simulink model "IFOCv6"  (R2022b)
settings: Solver=ode23tb  StartTime=0.0  StopTime=30  MaxStep=1e-5  RelTol=1e-4
InitFcn:
  | IFOCdatav6
values from neighbouring files (symbols this model uses):
  f_n = 300    [FOC_BANG_Script.m]    (also in IFOCdatav6.m)
  Im_n = k_im*Is_n    [FOC_BANG_Script.m]    (also in IFOCdatav6.m)
  Is_n = Pa/(3*Vsn_y*cos_phi)    [FOC_BANG_Script.m]    (also in IFOCdatav6.m)
  J = 5    [Data.m]    (also in FOC_BANG_Script.m; IFOCdatav6.m)
  ki_w = 0.5*(kp_w^2)/J    (= 3.92607044657)    [FOC_BANG_Script.m]    (also in IFOCdatav6.m = 613.448507277)
  kii = (1/2)*kpi^2/Ltot    [IFOCdatav6.m]
  kp_w = T_n/(0.05*wr_n)/5    (= 6.2658362942)    [FOC_BANG_Script.m]    (also in IFOCdatav6.m = 78.3229536775)
  kpi = (1/2)*Ltot/Ts    [IFOCdatav6.m]
  Lm = Phi_n/Im_n    [FOC_BANG_Script.m]    (also in IFOCdatav6.m)
  Lr = Ltot/2    [FOC_BANG_Script.m]    (also in IFOCdatav6.m)
  Ls = Ltot/2    [FOC_BANG_Script.m]    (also in IFOCdatav6.m)
  p = 6    [Data.m]    (also in FOC_BANG_Script.m; IFOCdatav6.m)
  P_n = 150000    [FOC_BANG_Script.m]    (also in IFOCdatav6.m)
  Rr = Rs    [FOC_BANG_Script.m]    (also in IFOCdatav6.m)
  Rs = (Pjs/3)/(Is_n^2)    [FOC_BANG_Script.m]    (also in IFOCdatav6.m)
  sigma_r = Lr/Lm    [FOC_BANG_Script.m]    (also in IFOCdatav6.m)
  sigma_s = Ls/Lm    [FOC_BANG_Script.m]    (also in IFOCdatav6.m)
  T_n = P_n/wr_n    (= 484.735867285)    [FOC_BANG_Script.m]    (also in IFOCdatav6.m)
  Tr = Lm*(1+sigma_r)/Rr    [FOC_BANG_Script.m]    (also in IFOCdatav6.m)
  Ts = 1/fs    (= 5e-05)    [FOC_BANG_Script.m]    (also in IFOCdatav6.m = 0.0001)
  Vdc = 350    [Data.m]    (also in FOC_BANG_Script.m; IFOCdatav6.m)
  Vs_n = 220    [FOC_BANG_Script.m]    (also in IFOCdatav6.m)
  Vsn_y = Vs_n/sqrt(3)    [FOC_BANG_Script.m]    (also in IFOCdatav6.m)
  wr_n = w_n/p*(1-s_n)    (= 309.446876379)    [FOC_BANG_Script.m]    (also in IFOCdatav6.m)
undefined symbols (not defined in the file or in its folder): DiscIntNeverNeededParam, sigbuilder_block
libraries: slpidlib x3, spsControlledVoltageSourceLib x3, spsCurrentMeasurementLib x3, eeTransforms x2, spsAsynchronousMachineSIUnitsLib x1, spsGroundLib x1, simulink x1, sps_lib x1
settings Model: Creator=39388  LastModifiedBy=v4pal
settings DebuggingCC: UnconnectedInputMsg=warning  UnconnectedOutputMsg=warning  UnconnectedLineMsg=warning  SFMachineParentedDataDiag=warning
settings ModelReferenceCC: EnableRefExpFcnMdlSchedulingChecks=on
settings RTWCC: DLArmComputeVersion=19.05

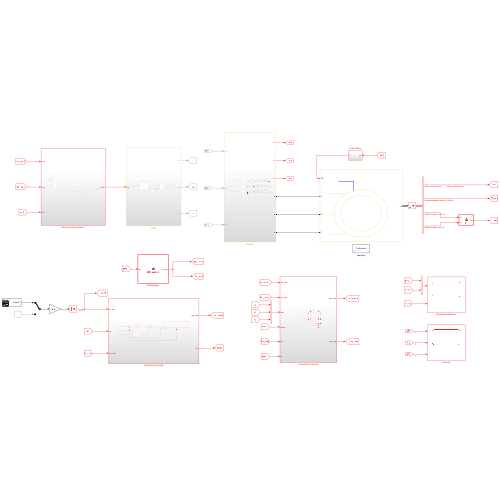
[thumbnail: Simulink's stored preview of the top-level diagram]
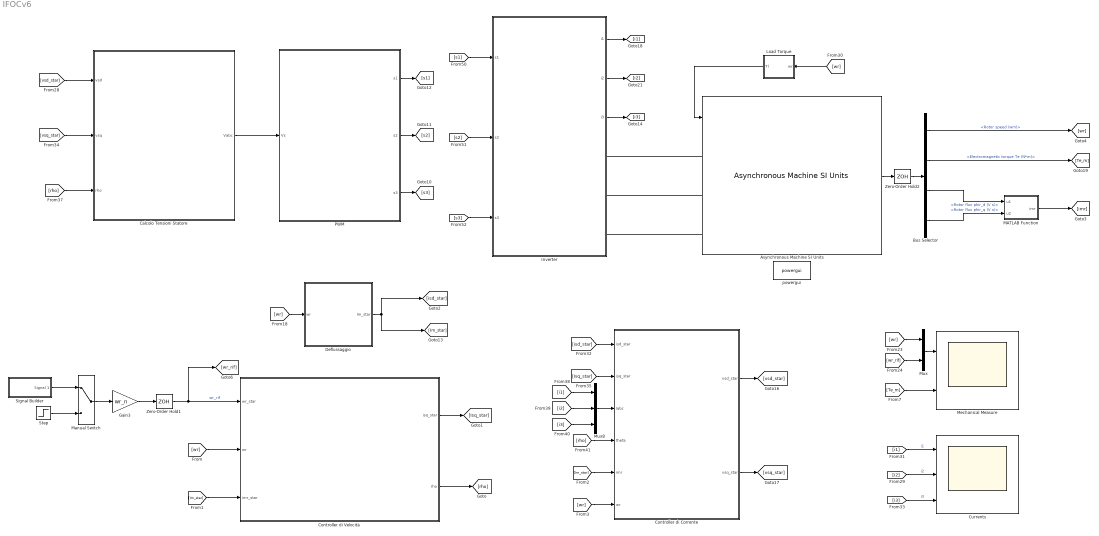
== system IFOCv6 ==
  Asynchronous Machine SI Units : spsAsynchronousMachineSIUnitsLib/Asynchronous Machine SI Units  RotorType=Squirrel-cage  PresetModel=No  MechanicalLoad=Torque Tm  ShowDetailedParameters=on  ReferenceFrame=Rotor  Units=SI  MeasurementBus=off  NominalParameters=[P_n Vs_n f_n]  VoltageRatio=1  Stator=[Rs Ls]  Rotor=[Rr Lr]  Cage1=[0.4155 0.002066]  Cage2=[0.4168 0.0003495]  Lm=Lm  Mechanical=[J 0 p]  PolePairs=2  InitialConditions=[1 0 0 0 0 0 0 0]  SimulateSaturation=off  Saturation=[14.03593122, 27.81365428, 53.79336849, 72.68890987, 97.98006896, 148.6815601, 215.7428561, 302.9841135, 428.7778367 ; 230, 322, 414, 460, 506, 552, 598, 644, 690]  LoadFlowParameters=1492000  TsPowergui=0  TsBlock=-1  IterativeModel=Trapezoidal non iterative  IterativeDiscreteModel=Trapezoidal non iterative  Pmec=1.492e+006
  Bus Selector : BusSelector  OutputSignals=Mechanical.Rotor speed (wm),Mechanical.Electromagnetic torque Te (N*m),Rotor measurements.Rotor flux phir_d (V s),Rotor measurements.Rotor flux phir_q (V s)
  "Calcolo Tensioni Statore " : Subsystem
  Controller di Corrente : Subsystem
  Controller di Velocità : Subsystem
  Currents : Scope  NumInputPorts=3
  Deflussaggio : MATLAB Function  TreatAsAtomicUnit=on
  Gain3 : Gain  Gain=wr_n
  Inverter : Subsystem
  Load Torque : Subsystem
  MATLAB Function : MATLAB Function  TreatAsAtomicUnit=on
  Manual Switch : ManualSwitch
  Mechanical Measure : Scope  NumInputPorts=2
  Mux : Mux  Inputs=2
  Mux8 : Mux  Inputs=3
  PWM : Subsystem
  Signal Builder : Subsystem  Tag=STV Subsys  LoadFcn=sigbuilder_block('load');  StartFcn=sigbuilder_block('start');  StopFcn=sigbuilder_block('stop');  ClipboardFcn=sigbuilder_block('clipboard');  mask(Sigbuilder block){tuvar=[0:10]}
      mask help: Simulink:masks:SigbuilderBlock_MD
      mask init:
      | if ~strcmp(get_param(bdroot(gcbh),'SimulationStatus'),'stopped') tuvar = sigbuilder_block('maskInit'); end
      settings: CopyFcn=sigbuilder_block('copy');  DeleteFcn=sigbuilder_block('delete');  ModelCloseFcn=sigbuilder_block('modelClose');  PreSaveFcn=sigbuilder_block('preSave');  PauseFcn=sigbuilder_block('pause');  ContinueFcn=sigbuilder_block('continue');  NameChangeFcn=sigbuilder_block('namechange');  OpenFcn=sigbuilder_block('open',[433.2 162 550.8 400.2 ]);  CloseFcn=sigbuilder_block('close');
      mask Display: plot(0, 0, 100, 100,[2, 2, 32, 32, 2], [68, 8, 8, 68, 68],[32, 2], [38, 38], [32, 19, 2],[53, 60, 44], [32, 17, 17, 2],[16, 16, 31, 31]);txt = getActiveGroup(gcbh);text(2, 100, txt,'verticalAlignment', 'top');
  Step : Step  Time=0  After=2  SampleTime=0
  Zero-Order Hold1 : ZeroOrderHold  SampleTime=Ts
  Zero-Order Hold2 : ZeroOrderHold  SampleTime=Ts
  powergui : sps_lib/powergui  Priority=1  SimulationMode=Continuous  SampleTime=50e-6  frequency=60  Iterations=50  frequencyindice=0  Pbase=100e6  ErrMax=1e-4  UnitsV=kV  UnitsW=MW  buscounter=0  FunctionMessages=off  echomessages=off  EnableUseOfTLC=off  CurrentSourceSwitches=off  DisableSnubberDevices=off  DisableRonSwitches=off  DisableVfSwitches=off  DisplayEquations=off  AutomaticDiscreteSolvers=off  SolverType=Tustin/Backward Euler (TBE)  Interpol=off  ExternalGateDelay=off  methode=off  Ts=100  x0status=blocks  SPID=on  SwTol=0  HookPort=off  NonlinearTolerance=1e-4  nMaxIteration=100  ContinueOnMaxIteration=off  RestoreLinks=warning  ResistiveCurrentMeasurement=off  Frange=[0:2:500]  Ylog=off  Xlog=on  ShowGrid=off  save=off  variable=ZData  structure=0  ZoomFFT=off  StartTime=0.0  cycles=1  DisplayStyle=1  fundamental=60  FreqAxis=off  MaxFrequency=1000  frequencyindicesteady=1  RmsSteady=1  display=off
  wires:
  Asynchronous Machine SI Units/1 -> Zero-Order Hold2/1
  Bus Selector/1 -> [wr]  "<Rotor speed (wm)>"
  [wr] -> Load Torque/1(wr)
  Load Torque/1(Tl) -> Asynchronous Machine SI Units/1
  [wr] -> Deflussaggio/1(wr)
  Zero-Order Hold1/1 -> [wr_rif], Controller di Velocità/1(wr_star)  "wr_rif"
  Gain3/1 -> Zero-Order Hold1/1
  Manual Switch/1 -> Gain3/1
  Signal Builder/1(Signal 1) -> Manual Switch/1
  Step/1 -> Manual Switch/2
  [i2] -> Currents/2  "i2"
  [i3] -> Currents/3  "i3"
  [i1] -> Currents/1  "i1"
  [i1] -> Mux8/1
  [i3] -> Mux8/3
  [i2] -> Mux8/2
  Bus Selector/2 -> [Te_m]  "<Electromagnetic torque Te (N*m)>"
  Deflussaggio/1(Im_star) -> [isd_star], [Im_star]
  PWM/1(s1) -> [s1]
  PWM/2(s2) -> [s2]
  PWM/3(s3) -> [s3]
  [vsd_star] -> "Calcolo Tensioni Statore "/1(vsd)
  [vsq_star] -> "Calcolo Tensioni Statore "/2(vsq)
  [rho] -> "Calcolo Tensioni Statore "/3(rho)
  [isd_star] -> Controller di Corrente/1(isd_star)
  [Isq_star] -> Controller di Corrente/2(isq_star)
  Mux8/1 -> Controller di Corrente/3(Iabc)
  [rho] -> Controller di Corrente/4(theta)
  Controller di Corrente/1(vsd_star) -> [vsd_star]
  Controller di Corrente/2(vsq_star) -> [vsq_star]
  [wr] -> Controller di Velocità/2(wr)
  [Im_star] -> Controller di Velocità/3(imr_star)
  Controller di Velocità/1(isq_star) -> [Isq_star]
  Controller di Velocità/2(rho) -> [rho]
  [s1] -> Inverter/1(s1)
  [s2] -> Inverter/2(s2)
  [s3] -> Inverter/3(s3)
  Inverter/1(i1) -> [i1]
  Inverter/2(i2) -> [i2]
  Inverter/3(i3) -> [i3]
  Bus Selector/3 -> MATLAB Function/1(u1)  "<Rotor flux phir_d (V s)>"
  Bus Selector/4 -> MATLAB Function/2(u2)  "<Rotor flux phir_q (V s)>"
  MATLAB Function/1(imr) -> [imr]
  "Calcolo Tensioni Statore "/1(Vabc) -> PWM/1(Vs)
  [Im_star] -> Controller di Corrente/5(imr)
  Zero-Order Hold2/1 -> Bus Selector/1
  [wr] -> Controller di Corrente/6(wr)
  [Te_m] -> Mechanical Measure/2
  Mux/1 -> Mechanical Measure/1
  [wr] -> Mux/1
  [wr_rif] -> Mux/2
  connections:
  Asynchronous Machine SI Units/LConn1 -- Inverter/RConn1
  Asynchronous Machine SI Units/LConn2 -- Inverter/RConn2
  Asynchronous Machine SI Units/LConn3 -- Inverter/RConn3

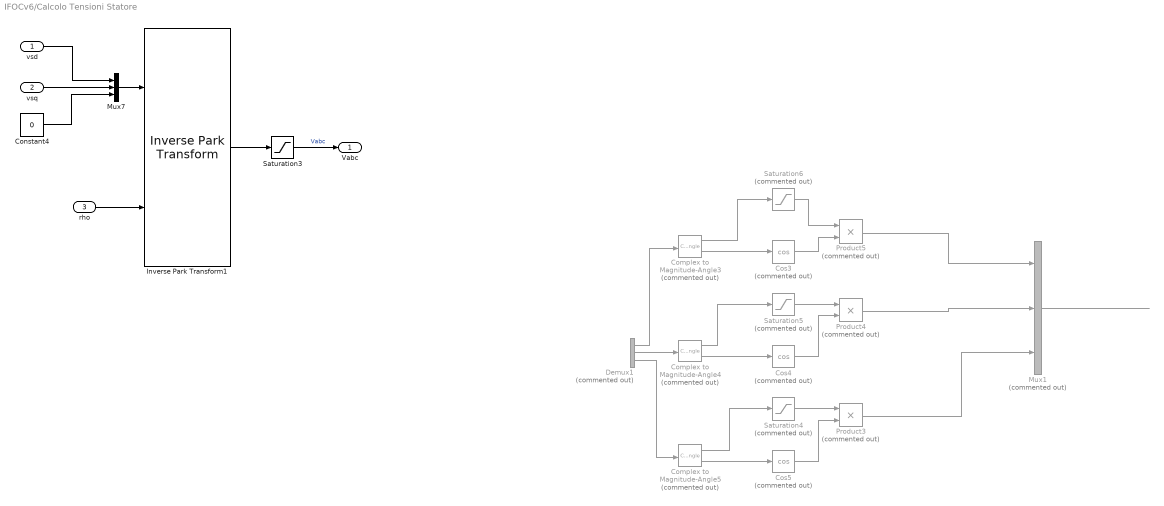
== system IFOCv6/Calcolo Tensioni Statore  ==
  vsd : Inport
  vsq : Inport  Port=2
  rho : Inport  Port=3
  Complex to Magnitude-Angle3 : ComplexToMagnitudeAngle  Commented=on
  Complex to Magnitude-Angle4 : ComplexToMagnitudeAngle  Commented=on
  Complex to Magnitude-Angle5 : ComplexToMagnitudeAngle  Commented=on
  Constant4 : Constant  Value=0
  Cos3 : Trigonometry  Commented=on  Operator=cos
  Cos4 : Trigonometry  Commented=on  Operator=cos
  Cos5 : Trigonometry  Commented=on  Operator=cos
  Demux1 : Demux  Commented=on  Outputs=3
  Inverse Park Transform1 : eeTransforms/Inverse Park Transform  AxisAlignment=Q-axis  PowerInvariant=off
      settings: LibrarySourceBlock=|
      | ee_sl_lib/Mathematical
      | Transforms/Inverse
      | Park Transform
  Mux1 : Mux  Commented=on  Inputs=3
  Mux7 : Mux  Inputs=3
  Product3 : Product  Commented=on
  Product4 : Product  Commented=on
  Product5 : Product  Commented=on
  Saturation3 : Saturate  UpperLimit=Vsn_y*sqrt(2)  LowerLimit=-Vsn_y*sqrt(2)
  Saturation4 : Saturate  Commented=on  UpperLimit=Vsn_y*sqrt(2)  LowerLimit=-Vsn_y*sqrt(2)
  Saturation5 : Saturate  Commented=on  UpperLimit=Vsn_y*sqrt(2)  LowerLimit=-Vsn_y*sqrt(2)
  Saturation6 : Saturate  Commented=on  UpperLimit=Vsn_y*sqrt(2)  LowerLimit=-Vsn_y*sqrt(2)
  Vabc : Outport
  wires:
  Mux7/1 -> Inverse Park Transform1/1
  Constant4/1 -> Mux7/3
  vsd/1 -> Mux7/1
  vsq/1 -> Mux7/2
  rho/1 -> Inverse Park Transform1/2
  Saturation6/1 -> Product5/1
  Saturation5/1 -> Product4/1
  Saturation4/1 -> Product3/1
  Complex to Magnitude-Angle5/1 -> Saturation4/1
  Complex to Magnitude-Angle3/1 -> Saturation6/1
  Cos3/1 -> Product5/2
  Complex to Magnitude-Angle4/1 -> Saturation5/1
  Cos4/1 -> Product4/2
  Cos5/1 -> Product3/2
  Complex to Magnitude-Angle5/2 -> Cos5/1
  Complex to Magnitude-Angle4/2 -> Cos4/1
  Complex to Magnitude-Angle3/2 -> Cos3/1
  Product3/1 -> Mux1/3
  Product4/1 -> Mux1/2
  Product5/1 -> Mux1/1
  Demux1/3 -> Complex to Magnitude-Angle5/1
  Demux1/2 -> Complex to Magnitude-Angle4/1
  Demux1/1 -> Complex to Magnitude-Angle3/1
  ? -> Demux1/1
  Mux1/1 -> ?
  Inverse Park Transform1/1 -> Saturation3/1
  Saturation3/1 -> Vabc/1  "Vabc"

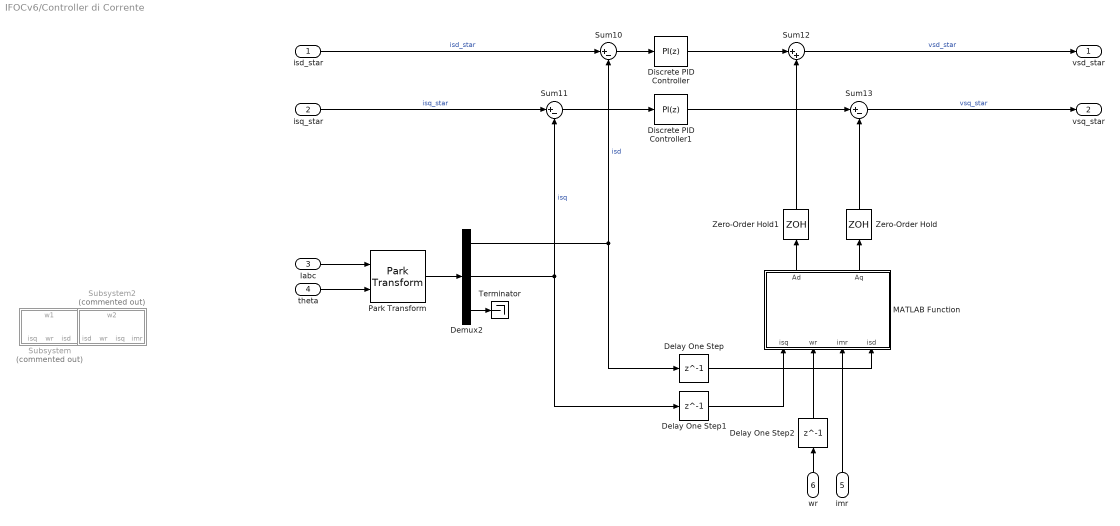
== system IFOCv6/Controller di Corrente ==
  isd_star : Inport
  isq_star : Inport  Port=2
  Iabc : Inport  Port=3
  theta : Inport  Port=4
  imr : Inport  Port=5
  wr : Inport  Port=6
  Delay One Step : Delay  DelayLength=1
  Delay One Step1 : Delay  DelayLength=1  InitialCondition=Im_n
  Delay One Step2 : Delay  DelayLength=1
  Demux2 : Demux  Outputs=3
  Discrete PID Controller : slpidlib/PID Controller  Controller=PI  Form=Parallel  TimeDomain=Discrete-time  UseExternalTs=off  SampleTime=Ts  IntegratorMethod=Forward Euler  FilterMethod=Forward Euler  ControllerParametersSource=internal  P=kpi  I=0.5*kii  UseKiTs=off  D=0  N=100  UseFilter=on  TunerSelectOption=Transfer Function Based (PID Tuner App)  InitialConditionSource=internal  InitialConditionForIntegrator=0  InitialConditionForFilter=0  DifferentiatorICPrevScaledInput=0  ExternalReset=none  TrackingMode=off  Kt=1  LimitOutput=on  SatLimitsSource=internal  UpperSaturationLimit=inf  LowerSaturationLimit=-inf  LinearizeAsGain=off  AntiWindupMode=clamping  Kb=1  LimitIntegrator=off  UpperIntegratorSaturationLimit=inf  LowerIntegratorSaturationLimit=-inf  POutMin=[]  POutMax=[]  IOutMin=[]  IOutMax=[]  DOutMin=[]  DOutMax=[]  NOutMin=[]  NOutMax=[]  SumOutMin=[]  SumOutMax=[]  SaturationOutMin=[]  SaturationOutMax=[]  PParamMin=[]  PParamMax=[]  IParamMin=[]  IParamMax=[]  DParamMin=[]  DParamMax=[]  NParamMin=[]  NParamMax=[]  KbParamMin=[]  KbParamMax=[]  KtParamMin=[]  KtParamMax=[]  KbOutMin=[]  KbOutMax=[]  KtOutMin=[]  KtOutMax=[]  IntegratorOutMin=[]  IntegratorOutMax=[]  FilterOutMin=[]  FilterOutMax=[]  SumI1OutMin=[]  SumI1OutMax=[]  SumI2OutMin=[]  SumI2OutMax=[]  SumI3OutMin=[]  SumI3OutMax=[]  SumI4OutMin=[]  SumI4OutMax=[]  SumDOutMin=[]  SumDOutMax=[]  DifferentiatorOutMin=[]  DifferentiatorOutMax=[]  FilterDiffOutCoefMin=[]  FilterDiffOutCoefMax=[]  ReciprocalOutMin=[]  ReciprocalOutMax=[]  SumDenOutMin=[]  SumDenOutMax=[]  SumNumOutMin=[]  SumNumOutMax=[]  DivideOutMin=[]  DivideOutMax=[]  UdiffTsProdOutMin=[]  UdiffTsProdOutMax=[]  NTsProdOutMin=[]  NTsProdOutMax=[]  UintegralTsProdOutMin=[]  UintegralTsProdOutMax=[]  UngainTsProdOutMin=[]  UngainTsProdOutMax=[]  ClampingZeroOutDataTypeStr=Inherit: Inherit via back propagation  ClampingZeroOutMin=[]  ClampingZeroOutMax=[]  FilterDenConstantOutDataTypeStr=Inherit: Inherit via back propagation  FilterDenConstantOutMin=[]  FilterDenConstantOutMax=[]  PCopyOutDataTypeStr=Inherit: Inherit via back propagation  PCopyOutMin=[]  PCopyOutMax=[]  NCopyOutDataTypeStr=Inherit: Inherit via back propagation  NCopyOutMin=[]  NCopyOutMax=[]  IntegratorContinuousStateAttributes=''  IntegratorStateMustResolveToSignalObject=off  IntegratorRTWStateStorageClass=Auto  FilterContinuousStateAttributes=''  FilterStateMustResolveToSignalObject=off  FilterRTWStateStorageClass=Auto  ParallelPVariant=InternalParameters  IdealPVariant=Disabled  IVariant=InternalParameters  DVariant=Disabled  IntegratorVariant=Discrete  SatVariant=Enabled  AWVariant=DiscClampingParallel  PCopyVariant=Disabled  TRVariant=Disabled  FdbkBlocksVariant=Forward  IdealPFdbkVariant=Disabled  SatFdbkVariant=Disabled  DerivativeFilterVariant=Disabled  NVariant=Disabled  NCopyVariant=Disabled_SignalSpec  FilterICVariant=Disabled  IntegratorICVariant=InternalICs  ExternalResetVariant=Disabled  TRSumVariant=Passthrough  SumFdbkVariant=Disabled  SumVariant=Sum_PI  TsampFilterVariant=InternalTs  TsampNgainVariant=Passthrough  TsampIntegralVariant=Passthrough  ExternalSaturationOutDataTypeStr=Inherit: Same as second input
      settings: LibrarySourceBlock=simulink/Discrete/Discrete PID Controller
  Discrete PID Controller1 : slpidlib/PID Controller  Controller=PI  Form=Parallel  TimeDomain=Discrete-time  UseExternalTs=off  SampleTime=Ts  IntegratorMethod=Forward Euler  FilterMethod=Forward Euler  ControllerParametersSource=internal  P=kpi  I=0.5*kii  UseKiTs=off  D=0  N=100  UseFilter=on  TunerSelectOption=Transfer Function Based (PID Tuner App)  InitialConditionSource=internal  InitialConditionForIntegrator=0  InitialConditionForFilter=0  DifferentiatorICPrevScaledInput=0  ExternalReset=none  TrackingMode=off  Kt=1  LimitOutput=on  SatLimitsSource=internal  UpperSaturationLimit=inf  LowerSaturationLimit=-inf  LinearizeAsGain=off  AntiWindupMode=clamping  Kb=1  LimitIntegrator=off  UpperIntegratorSaturationLimit=inf  LowerIntegratorSaturationLimit=-inf  POutMin=[]  POutMax=[]  IOutMin=[]  IOutMax=[]  DOutMin=[]  DOutMax=[]  NOutMin=[]  NOutMax=[]  SumOutMin=[]  SumOutMax=[]  SaturationOutMin=[]  SaturationOutMax=[]  PParamMin=[]  PParamMax=[]  IParamMin=[]  IParamMax=[]  DParamMin=[]  DParamMax=[]  NParamMin=[]  NParamMax=[]  KbParamMin=[]  KbParamMax=[]  KtParamMin=[]  KtParamMax=[]  KbOutMin=[]  KbOutMax=[]  KtOutMin=[]  KtOutMax=[]  IntegratorOutMin=[]  IntegratorOutMax=[]  FilterOutMin=[]  FilterOutMax=[]  SumI1OutMin=[]  SumI1OutMax=[]  SumI2OutMin=[]  SumI2OutMax=[]  SumI3OutMin=[]  SumI3OutMax=[]  SumI4OutMin=[]  SumI4OutMax=[]  SumDOutMin=[]  SumDOutMax=[]  DifferentiatorOutMin=[]  DifferentiatorOutMax=[]  FilterDiffOutCoefMin=[]  FilterDiffOutCoefMax=[]  ReciprocalOutMin=[]  ReciprocalOutMax=[]  SumDenOutMin=[]  SumDenOutMax=[]  SumNumOutMin=[]  SumNumOutMax=[]  DivideOutMin=[]  DivideOutMax=[]  UdiffTsProdOutMin=[]  UdiffTsProdOutMax=[]  NTsProdOutMin=[]  NTsProdOutMax=[]  UintegralTsProdOutMin=[]  UintegralTsProdOutMax=[]  UngainTsProdOutMin=[]  UngainTsProdOutMax=[]  ClampingZeroOutDataTypeStr=Inherit: Inherit via back propagation  ClampingZeroOutMin=[]  ClampingZeroOutMax=[]  FilterDenConstantOutDataTypeStr=Inherit: Inherit via back propagation  FilterDenConstantOutMin=[]  FilterDenConstantOutMax=[]  PCopyOutDataTypeStr=Inherit: Inherit via back propagation  PCopyOutMin=[]  PCopyOutMax=[]  NCopyOutDataTypeStr=Inherit: Inherit via back propagation  NCopyOutMin=[]  NCopyOutMax=[]  IntegratorContinuousStateAttributes=''  IntegratorStateMustResolveToSignalObject=off  IntegratorRTWStateStorageClass=Auto  FilterContinuousStateAttributes=''  FilterStateMustResolveToSignalObject=off  FilterRTWStateStorageClass=Auto  ParallelPVariant=InternalParameters  IdealPVariant=Disabled  IVariant=InternalParameters  DVariant=Disabled  IntegratorVariant=Discrete  SatVariant=Enabled  AWVariant=DiscClampingParallel  PCopyVariant=Disabled  TRVariant=Disabled  FdbkBlocksVariant=Forward  IdealPFdbkVariant=Disabled  SatFdbkVariant=Disabled  DerivativeFilterVariant=Disabled  NVariant=Disabled  NCopyVariant=Disabled_SignalSpec  FilterICVariant=Disabled  IntegratorICVariant=InternalICs  ExternalResetVariant=Disabled  TRSumVariant=Passthrough  SumFdbkVariant=Disabled  SumVariant=Sum_PI  TsampFilterVariant=InternalTs  TsampNgainVariant=Passthrough  TsampIntegralVariant=Passthrough  ExternalSaturationOutDataTypeStr=Inherit: Same as second input
      settings: LibrarySourceBlock=simulink/Discrete/Discrete PID Controller
  MATLAB Function : MATLAB Function  TreatAsAtomicUnit=on
  Park Transform : eeTransforms/Park Transform  AxisAlignment=Q-axis  PowerInvariant=off
      settings: LibrarySourceBlock=|
      | ee_sl_lib/Mathematical
      | Transforms/Park Transform
  Subsystem : Subsystem  Commented=on
  Subsystem2 : Subsystem  Commented=on
  Sum10 : Sum  Inputs=|+-
  Sum11 : Sum  Inputs=|+-
  Sum12 : Sum  Inputs=|++
  Sum13 : Sum  Inputs=|+-
  Terminator : Terminator
  Zero-Order Hold : ZeroOrderHold  SampleTime=-1
  Zero-Order Hold1 : ZeroOrderHold  SampleTime=-1
  vsd_star : Outport
  vsq_star : Outport  Port=2
  wires:
  Sum13/1 -> vsq_star/1  "vsq_star"
  Park Transform/1 -> Demux2/1
  Demux2/2 -> Delay One Step1/1, Sum11/2  "isq"
  Demux2/1 -> Delay One Step/1, Sum10/2  "isd"
  Sum12/1 -> vsd_star/1  "vsd_star"
  Sum10/1 -> Discrete PID Controller/1
  Sum11/1 -> Discrete PID Controller1/1
  Demux2/3 -> Terminator/1
  isq_star/1 -> Sum11/1  "isq_star"
  theta/1 -> Park Transform/2
  Iabc/1 -> Park Transform/1
  isd_star/1 -> Sum10/1  "isd_star"
  Discrete PID Controller1/1 -> Sum13/1
  Discrete PID Controller/1 -> Sum12/1
  Zero-Order Hold/1 -> Sum13/2
  Zero-Order Hold1/1 -> Sum12/2
  MATLAB Function/2(Aq) -> Zero-Order Hold/1
  MATLAB Function/1(Ad) -> Zero-Order Hold1/1
  Delay One Step/1 -> MATLAB Function/4(isd)
  Delay One Step1/1 -> MATLAB Function/1(isq)
  Delay One Step2/1 -> MATLAB Function/2(wr)
  imr/1 -> MATLAB Function/3(imr)
  wr/1 -> Delay One Step2/1

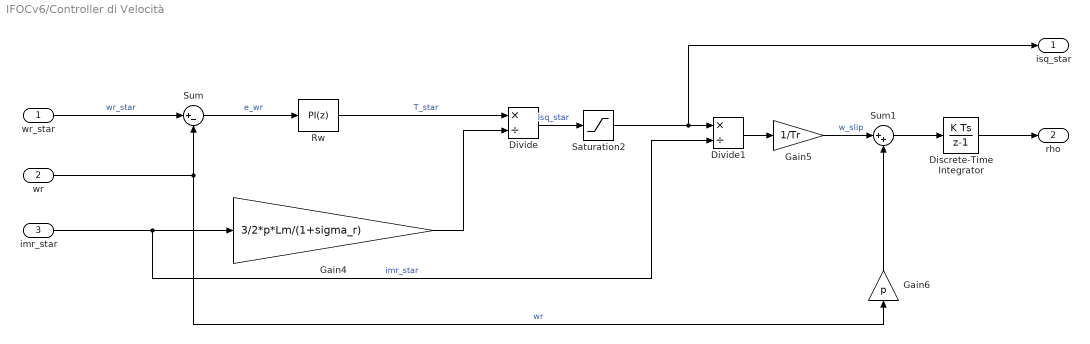
== system IFOCv6/Controller di Velocità ==
  wr_star : Inport
  wr : Inport  Port=2
  imr_star : Inport  Port=3
  Discrete-Time Integrator : DiscreteIntegrator  SampleTime=Ts  ICPrevOutput=DiscIntNeverNeededParam  ICPrevScaledInput=DiscIntNeverNeededParam
  Divide : Product  Inputs=*/
  Divide1 : Product  Inputs=*/
  Gain4 : Gain  Gain=3/2*p*Lm/(1+sigma_r)
  Gain5 : Gain  Gain=1/Tr
  Gain6 : Gain  Gain=p
  Rw : slpidlib/PID Controller  Controller=PI  Form=Parallel  TimeDomain=Discrete-time  UseExternalTs=off  SampleTime=Ts  IntegratorMethod=Trapezoidal  FilterMethod=Forward Euler  ControllerParametersSource=internal  P=kp_w  I=ki_w  UseKiTs=off  D=0  N=100  UseFilter=on  TunerSelectOption=Frequency Response Based  InitialConditionSource=internal  InitialConditionForIntegrator=0  InitialConditionForFilter=0  DifferentiatorICPrevScaledInput=0  ExternalReset=none  TrackingMode=off  Kt=1  LimitOutput=on  SatLimitsSource=internal  UpperSaturationLimit=T_n  LowerSaturationLimit=-T_n  LinearizeAsGain=on  AntiWindupMode=clamping  Kb=1  LimitIntegrator=off  UpperIntegratorSaturationLimit=inf  LowerIntegratorSaturationLimit=-inf  POutMin=[]  POutMax=[]  IOutMin=[]  IOutMax=[]  DOutMin=[]  DOutMax=[]  NOutMin=[]  NOutMax=[]  SumOutMin=[]  SumOutMax=[]  SaturationOutMin=[]  SaturationOutMax=[]  PParamMin=[]  PParamMax=[]  IParamMin=[]  IParamMax=[]  DParamMin=[]  DParamMax=[]  NParamMin=[]  NParamMax=[]  KbParamMin=[]  KbParamMax=[]  KtParamMin=[]  KtParamMax=[]  KbOutMin=[]  KbOutMax=[]  KtOutMin=[]  KtOutMax=[]  IntegratorOutMin=[]  IntegratorOutMax=[]  FilterOutMin=[]  FilterOutMax=[]  SumI1OutMin=[]  SumI1OutMax=[]  SumI2OutMin=[]  SumI2OutMax=[]  SumI3OutMin=[]  SumI3OutMax=[]  SumI4OutMin=[]  SumI4OutMax=[]  SumDOutMin=[]  SumDOutMax=[]  DifferentiatorOutMin=[]  DifferentiatorOutMax=[]  FilterDiffOutCoefMin=[]  FilterDiffOutCoefMax=[]  ReciprocalOutMin=[]  ReciprocalOutMax=[]  SumDenOutMin=[]  SumDenOutMax=[]  SumNumOutMin=[]  SumNumOutMax=[]  DivideOutMin=[]  DivideOutMax=[]  UdiffTsProdOutMin=[]  UdiffTsProdOutMax=[]  NTsProdOutMin=[]  NTsProdOutMax=[]  UintegralTsProdOutMin=[]  UintegralTsProdOutMax=[]  UngainTsProdOutMin=[]  UngainTsProdOutMax=[]  ClampingZeroOutDataTypeStr=Inherit: Inherit via back propagation  ClampingZeroOutMin=[]  ClampingZeroOutMax=[]  FilterDenConstantOutDataTypeStr=Inherit: Inherit via back propagation  FilterDenConstantOutMin=[]  FilterDenConstantOutMax=[]  PCopyOutDataTypeStr=Inherit: Inherit via back propagation  PCopyOutMin=[]  PCopyOutMax=[]  NCopyOutDataTypeStr=Inherit: Inherit via back propagation  NCopyOutMin=[]  NCopyOutMax=[]  IntegratorContinuousStateAttributes=''  IntegratorStateMustResolveToSignalObject=off  IntegratorRTWStateStorageClass=Auto  FilterContinuousStateAttributes=''  FilterStateMustResolveToSignalObject=off  FilterRTWStateStorageClass=Auto  ParallelPVariant=InternalParameters  IdealPVariant=Disabled  IVariant=InternalParameters  DVariant=Disabled  IntegratorVariant=Discrete  SatVariant=Enabled  AWVariant=DiscClampingParallel  PCopyVariant=Disabled  TRVariant=Disabled  FdbkBlocksVariant=Feedback  IdealPFdbkVariant=Passthrough  SatFdbkVariant=Passthrough  DerivativeFilterVariant=Disabled  NVariant=Disabled  NCopyVariant=Disabled_SignalSpec  FilterICVariant=Disabled  IntegratorICVariant=InternalICs  ExternalResetVariant=Disabled  TRSumVariant=Passthrough  SumFdbkVariant=Enabled  SumVariant=Sum_PI  TsampFilterVariant=InternalTs  TsampNgainVariant=Passthrough  TsampIntegralVariant=Passthrough  ExternalSaturationOutDataTypeStr=Inherit: Same as second input
  Saturation2 : Saturate  UpperLimit=0.96*Is_n*sqrt(2)  LowerLimit=-0.96*Is_n*sqrt(2)
  Sum : Sum  Inputs=|+-
  Sum1 : Sum  Inputs=|++
  isq_star : Outport
  rho : Outport  Port=2
  wires:
  Sum1/1 -> Discrete-Time Integrator/1
  Divide1/1 -> Gain5/1
  Gain5/1 -> Sum1/1  "w_slip"
  Gain6/1 -> Sum1/2
  wr/1 -> Gain6/1, Sum/2  "wr"
  Sum/1 -> Rw/1  "e_wr"
  Rw/1 -> Divide/1  "T_star"
  Gain4/1 -> Divide/2
  Divide/1 -> Saturation2/1  "Isq_star"
  wr_star/1 -> Sum/1  "wr_star"
  Discrete-Time Integrator/1 -> rho/1
  imr_star/1 -> Divide1/2, Gain4/1  "imr_star"
  Saturation2/1 -> isq_star/1, Divide1/1

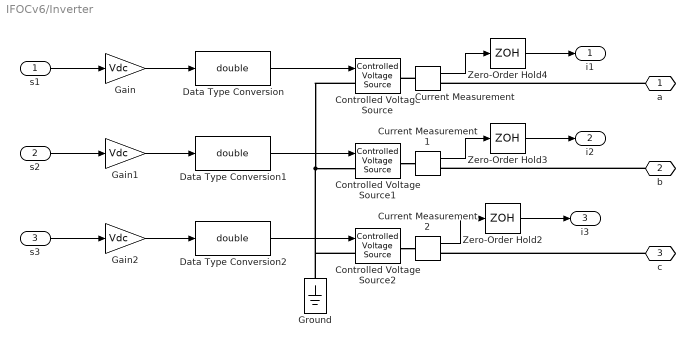
== system IFOCv6/Inverter ==
  s1 : Inport
  s2 : Inport  Port=2
  s3 : Inport  Port=3
  Controlled Voltage Source : spsControlledVoltageSourceLib/Controlled Voltage Source  Initialize=on  Source_Type=AC  Amplitude=0  Phase=0  Frequency=0  Measurements=None
  Controlled Voltage Source1 : spsControlledVoltageSourceLib/Controlled Voltage Source  Initialize=on  Source_Type=AC  Amplitude=0  Phase=0  Frequency=0  Measurements=None
  Controlled Voltage Source2 : spsControlledVoltageSourceLib/Controlled Voltage Source  Initialize=on  Source_Type=AC  Amplitude=0  Phase=0  Frequency=0  Measurements=None
  Current Measurement : spsCurrentMeasurementLib/Current Measurement  PhasorSimulation=off  OutputType=Complex  PSBequivalent=0
  Current Measurement1 : spsCurrentMeasurementLib/Current Measurement  PhasorSimulation=off  OutputType=Complex  PSBequivalent=0
  Current Measurement2 : spsCurrentMeasurementLib/Current Measurement  PhasorSimulation=off  OutputType=Complex  PSBequivalent=0
  Data Type Conversion : DataTypeConversion  OutDataTypeStr=double  SaturateOnIntegerOverflow=off  RndMeth=Floor
  Data Type Conversion1 : DataTypeConversion  OutDataTypeStr=double  SaturateOnIntegerOverflow=off  RndMeth=Floor
  Data Type Conversion2 : DataTypeConversion  OutDataTypeStr=double  SaturateOnIntegerOverflow=off  RndMeth=Floor
  Gain : Gain  Gain=Vdc
  Gain1 : Gain  Gain=Vdc
  Gain2 : Gain  Gain=Vdc
  Ground : spsGroundLib/Ground  LConnTagsString=a
  Zero-Order Hold2 : ZeroOrderHold  SampleTime=Ts
  Zero-Order Hold3 : ZeroOrderHold  SampleTime=Ts
  Zero-Order Hold4 : ZeroOrderHold  SampleTime=Ts
  a : PMIOPort  Side=Right
  b : PMIOPort  Port=2  Side=Right
  c : PMIOPort  Port=3  Side=Right
  i1 : Outport
  i2 : Outport  Port=2
  i3 : Outport  Port=3
  wires:
  Gain/1 -> Data Type Conversion/1
  Zero-Order Hold4/1 -> i1/1
  Gain1/1 -> Data Type Conversion1/1
  Current Measurement2/1 -> Zero-Order Hold2/1
  Current Measurement/1 -> Zero-Order Hold4/1
  Gain2/1 -> Data Type Conversion2/1
  Current Measurement1/1 -> Zero-Order Hold3/1
  Data Type Conversion1/1 -> Controlled Voltage Source1/1
  Data Type Conversion2/1 -> Controlled Voltage Source2/1
  s3/1 -> Gain2/1
  Data Type Conversion/1 -> Controlled Voltage Source/1
  s2/1 -> Gain1/1
  Zero-Order Hold2/1 -> i3/1
  Zero-Order Hold3/1 -> i2/1
  s1/1 -> Gain/1
  connections:
  Controlled Voltage Source/LConn1 -- Ground/LConn1 -- Controlled Voltage Source2/LConn1 -- Controlled Voltage Source1/LConn1
  Controlled Voltage Source1/RConn1 -- Current Measurement1/LConn1
  Controlled Voltage Source2/RConn1 -- Current Measurement2/LConn1
  Current Measurement/LConn1 -- Controlled Voltage Source/RConn1
  b/RConn1 -- Current Measurement1/RConn1
  a/RConn1 -- Current Measurement/RConn1
  c/RConn1 -- Current Measurement2/RConn1

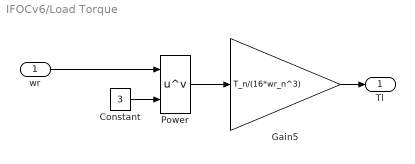
== system IFOCv6/Load Torque ==
  wr : Inport
  Constant : Constant  Value=3
  Gain5 : Gain  Gain=T_n/(16*wr_n^3)
  Power : Math  Operator=pow
  Tl : Outport
  wires:
  Power/1 -> Gain5/1
  Constant/1 -> Power/2
  Gain5/1 -> Tl/1
  wr/1 -> Power/1

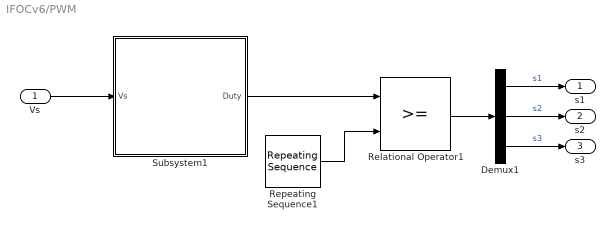
== system IFOCv6/PWM ==
  Vs : Inport
  Demux1 : Demux  Outputs=3
  Relational Operator1 : RelationalOperator  OutDataTypeStr=boolean  RndMeth=Simplest  InputSameDT=off
  Repeating Sequence1 : simulink/Sources/Repeating Sequence  rep_seq_t=[0 Ts/2 Ts]  rep_seq_y=[0 1 0]
  Subsystem1 : Subsystem
  s1 : Outport
  s2 : Outport  Port=2
  s3 : Outport  Port=3
  wires:
  Vs/1 -> Subsystem1/1(Vs)
  Subsystem1/1(Duty) -> Relational Operator1/1
  Repeating Sequence1/1 -> Relational Operator1/2
  Demux1/3 -> s3/1  "s3"
  Demux1/2 -> s2/1  "s2"
  Relational Operator1/1 -> Demux1/1
  Demux1/1 -> s1/1  "s1"

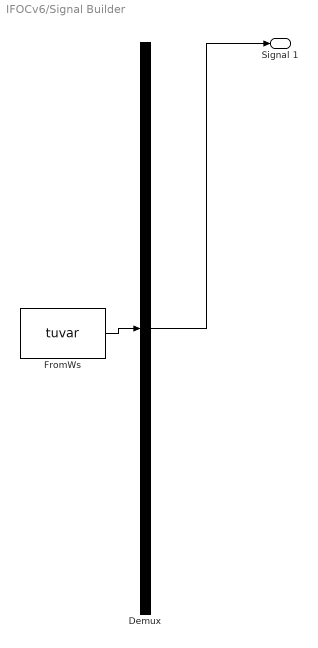
== system IFOCv6/Signal Builder ==
  Demux : Demux  Tag=STV Demux  Outputs=1
      settings: DisplayOption=none
  FromWs : FromWorkspace  Tag=STV FromWs  VariableName=tuvar
      SigBuilderData=|
      | common.afterFinalStr = 'Extrapolate'
      | common.sampleTime = 0
      | dataSet.timeRange = [0 30]
      | dataSet.name = 'Group 1'
      | sbobj.Groups.Name = 'Group 1'
      | sbobj.Groups.Signals.Name = 'Signal 1'
      | sbobj.Groups.Signals.XData = [0 0.2 0.2 5 10 20 25 30]
      | sbobj.Groups.Signals.YData = [0 0 1 1 2 2 1 1]
      | sbobj.Groups.TimeRange = [0 30]
  Signal 1 : Outport  Tag=STV Outport
  wires:
  Demux/1 -> Signal 1/1
  FromWs/1 -> Demux/1

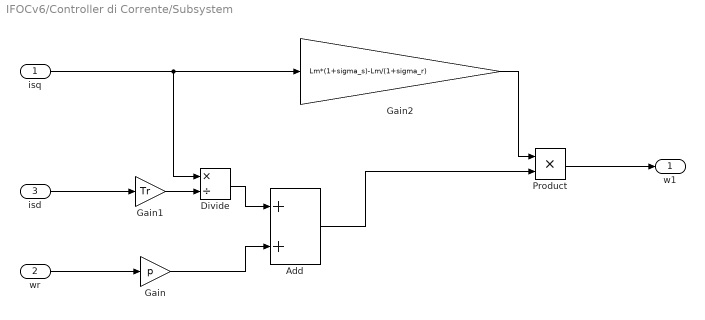
== system IFOCv6/Controller di Corrente/Subsystem ==
  isq : Inport
  wr : Inport  Port=2
  isd : Inport  Port=3
  Add : Sum
  Divide : Product  Inputs=*/
  Gain : Gain  Gain=p
  Gain1 : Gain  Gain=Tr
  Gain2 : Gain  Gain=Lm*(1+sigma_s)-Lm/(1+sigma_r)
  Product : Product
  w1 : Outport
  wires:
  wr/1 -> Gain/1
  Gain/1 -> Add/2
  isq/1 -> Divide/1, Gain2/1
  isd/1 -> Gain1/1
  Divide/1 -> Add/1
  Gain1/1 -> Divide/2
  Add/1 -> Product/2
  Product/1 -> w1/1
  Gain2/1 -> Product/1

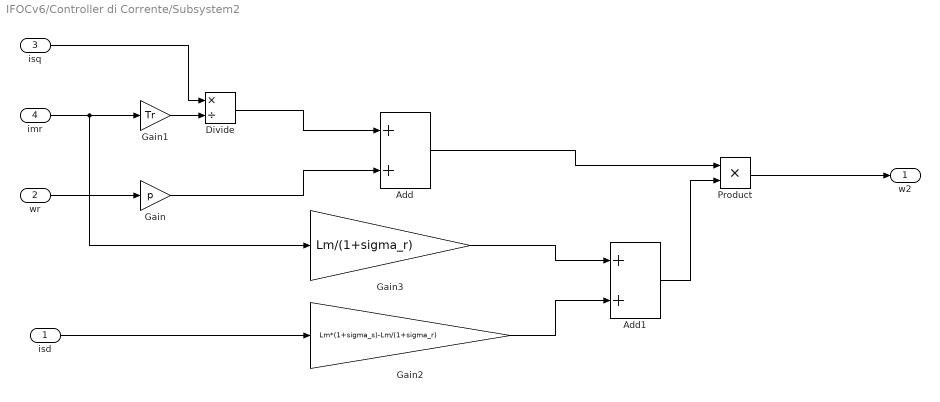
== system IFOCv6/Controller di Corrente/Subsystem2 ==
  isd : Inport
  wr : Inport  Port=2
  isq : Inport  Port=3
  imr : Inport  Port=4
  Add : Sum
  Add1 : Sum
  Divide : Product  Inputs=*/
  Gain : Gain  Gain=p
  Gain1 : Gain  Gain=Tr
  Gain2 : Gain  Gain=Lm*(1+sigma_s)-Lm/(1+sigma_r)
  Gain3 : Gain  Gain=Lm/(1+sigma_r)
  Product : Product
  w2 : Outport
  wires:
  Gain/1 -> Add/2
  Gain1/1 -> Divide/2
  Divide/1 -> Add/1
  wr/1 -> Gain/1
  isq/1 -> Divide/1
  Gain2/1 -> Add1/2
  Gain3/1 -> Add1/1
  Add1/1 -> Product/2
  Add/1 -> Product/1
  Product/1 -> w2/1
  imr/1 -> Gain3/1, Gain1/1
  isd/1 -> Gain2/1

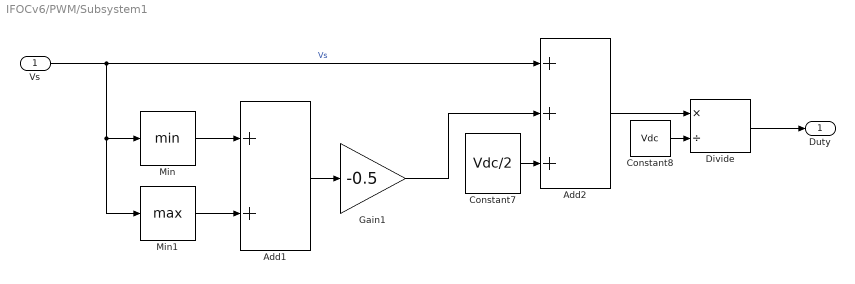
== system IFOCv6/PWM/Subsystem1 ==
  Vs : Inport  SampleTime=Ts
  Add1 : Sum
  Add2 : Sum  Inputs=+++
  Constant7 : Constant  Value=Vdc/2
  Constant8 : Constant  Value=Vdc
  Divide : Product  Inputs=*/  RndMeth=Zero  SaturateOnIntegerOverflow=on
  Gain1 : Gain  Gain=-0.5
  Min : MinMax
  Min1 : MinMax  Function=max
  Duty : Outport
  wires:
  Min1/1 -> Add1/2
  Gain1/1 -> Add2/2
  Divide/1 -> Duty/1
  Add1/1 -> Gain1/1
  Constant8/1 -> Divide/2
  Vs/1 -> Add2/1, Min/1, Min1/1  "Vs"
  Min/1 -> Add1/1
  Add2/1 -> Divide/1
  Constant7/1 -> Add2/3

== matlab function IFOCv6/MATLAB Function ==
  data: u1 input; imr output; u2 input; Lm parameter
function imr = fcn(u1,u2, Lm)

phi = sqrt(u1^(2)+u2^(2));
imr = phi/Lm;
end

== matlab function IFOCv6/Controller di Corrente/MATLAB Function ==
  data: Ad output; isq input; wr input; imr input; isd input; Aq output; p parameter; Tr parameter; sigma_r parameter; sigma_s parameter; Lm parameter
function [Ad, Aq] = decoupling(isq, wr, imr, isd, p, Tr, sigma_r, sigma_s, Lm)

delta = Lm*(1+sigma_s) - Lm/(1+sigma_r);

Ad = delta*isq*(p*wr + isq/Tr/imr) + Lm/(1+sigma_r)*(isd-imr)/Tr;

Aq = (p*wr + isq/Tr/imr) * (delta*isd + imr*Lm/(1+sigma_r));

== matlab function IFOCv6/Deflussaggio ==
  data: Im_star output; wr input; wr_n parameter; Im_n parameter
function Im_star = deflussaggio(wr, wr_n, Im_n)
k = Im_n*wr_n;

if wr > wr_n
    Im_star = k/((sqrt(wr_n))*(sqrt(wr)));
    %Im_star = k/wr;
else if wr < -wr_n
    Im_star = -k/((sqrt(wr_n))*(sqrt(wr)));
    %Im_star = -k/wr;
    else
    Im_star = Im_n;
end
end
end
